simulink model "natural_freq_of_rlc_11"  (R2018a)
settings: Solver=VariableStepAuto  StartTime=0.0  StopTime=2  RelTol=1e-3
settings Model: Creator=barne  LastModifiedBy=weishij2

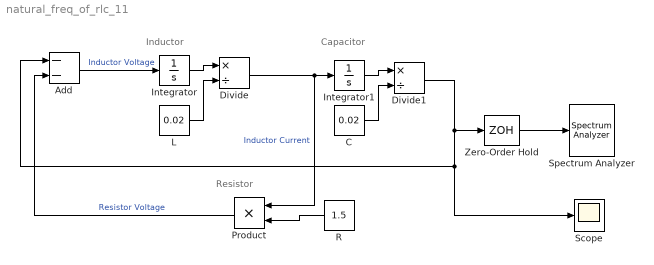
== system natural_freq_of_rlc_11 ==
  note: Resistor
  note: Inductor
  note: Capacitor
  Add : Sum  Inputs=--
  C : Constant  Value=0.02
  Divide : Product  Inputs=*/
  Divide1 : Product  Inputs=*/
  Integrator : Integrator  InitialCondition=0.1
  Integrator1 : Integrator  InitialCondition=0.1
  L : Constant  Value=0.02
  Product : Product
  R : Constant  Value=1.5
  Scope : Scope
  Spectrum Analyzer : SpectrumAnalyzer
  Zero-Order Hold : ZeroOrderHold  SampleTime=2^(-10)
  wires:
  Add/1 -> Integrator/1  "Inductor Voltage"
  Integrator/1 -> Divide/1
  L/1 -> Divide/2
  Divide/1 -> Product/1, Integrator1/1  "Inductor Current"
  Integrator1/1 -> Divide1/1
  C/1 -> Divide1/2
  R/1 -> Product/2
  Product/1 -> Add/2  "Resistor Voltage"
  Divide1/1 -> Scope/1, Add/1, Zero-Order Hold/1
  Zero-Order Hold/1 -> Spectrum Analyzer/1
